simulink library "Filter"  (R2018b)
settings: Solver=VariableStepAuto  StartTime=0.0  StopTime=10.0  RelTol=1e-3
undefined symbols (not defined in the file): DiscIntNeverNeededParam
settings Model: Creator=zouji  LastModifiedBy=zouji

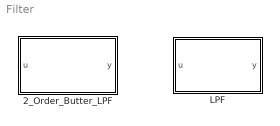
== system Filter ==
  2_Order_Butter_LPF : Subsystem  mask{wn=30*2*pi, ksi=0.707}
      mask prompts: wn "Cut Frequency (rad/s)"; ksi "Damping Ratio"
  LPF : Subsystem  mask{T=0.5}
      mask prompts: T "Time Constant"

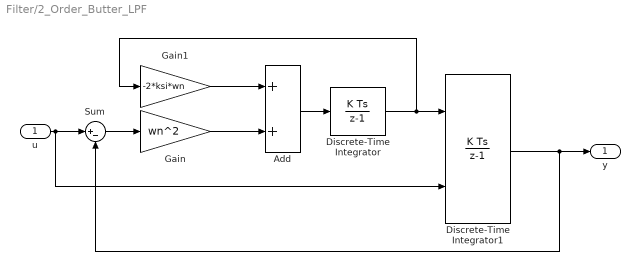
== system Filter/2_Order_Butter_LPF ==
  u : Inport
  Add : Sum
  Discrete-Time Integrator : DiscreteIntegrator  SampleTime=-1  ICPrevOutput=DiscIntNeverNeededParam  ICPrevScaledInput=DiscIntNeverNeededParam
  Discrete-Time Integrator1 : DiscreteIntegrator  InitialConditionSource=external  SampleTime=-1  ICPrevOutput=DiscIntNeverNeededParam  ICPrevScaledInput=DiscIntNeverNeededParam
  Gain : Gain  Gain=wn^2
  Gain1 : Gain  Gain=-2*ksi*wn
  Sum : Sum  Inputs=|+-
  y : Outport
  wires:
  Gain1/1 -> Add/1
  Add/1 -> Discrete-Time Integrator/1
  Sum/1 -> Gain/1
  Gain/1 -> Add/2
  Discrete-Time Integrator1/1 -> Sum/2, y/1
  Discrete-Time Integrator/1 -> Gain1/1, Discrete-Time Integrator1/1
  u/1 -> Discrete-Time Integrator1/2, Sum/1

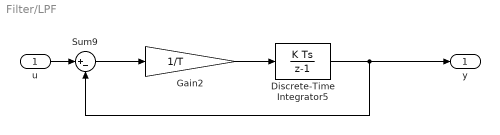
== system Filter/LPF ==
  u : Inport
  Discrete-Time Integrator5 : DiscreteIntegrator  SampleTime=-1  OutDataTypeStr=single  UpperSaturationLimit=20/180*pi  LowerSaturationLimit=-20/180*pi  ICPrevOutput=DiscIntNeverNeededParam  ICPrevScaledInput=DiscIntNeverNeededParam
  Gain2 : Gain  Gain=1/T
  Sum9 : Sum  Inputs=|+-
  y : Outport
  wires:
  u/1 -> Sum9/1
  Sum9/1 -> Gain2/1
  Discrete-Time Integrator5/1 -> y/1, Sum9/2
  Gain2/1 -> Discrete-Time Integrator5/1
